simulink model "Res_16"  (R2018b)
settings: Solver=VariableStepAuto  StartTime=0.0  StopTime=0.2  RelTol=1e-3
settings Model: Creator=makha  LastModifiedBy=makha

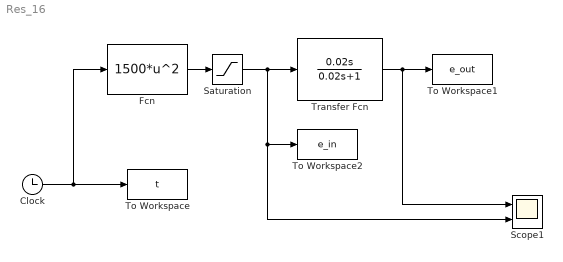
== system Res_16 ==
  Clock : Clock
  Fcn : Fcn  Expr=1500*u^2
  Saturation : Saturate  UpperLimit=2.4
  Scope1 : Scope  NumInputPorts=2
  To Workspace : ToWorkspace  VariableName=t  SampleTime=-1
  To Workspace1 : ToWorkspace  VariableName=e_out  SampleTime=-1
  To Workspace2 : ToWorkspace  VariableName=e_in  SampleTime=-1
  Transfer Fcn : TransferFcn  Numerator=[0.02 0]  Denominator=[0.02 1]
  wires:
  Clock/1 -> Fcn/1, To Workspace/1
  Saturation/1 -> Scope1/2, To Workspace2/1, Transfer Fcn/1
  Fcn/1 -> Saturation/1
  Transfer Fcn/1 -> Scope1/1, To Workspace1/1
